simulink model "KUKA_PRRR"  (R2021a)
settings: Solver=FixedStepAuto  StartTime=0.0  StopTime=1  FixedStep=0.001  RelTol=1e-3
values from neighbouring files (symbols this model uses):
  m = {0 0 0 0 0}    [DynMatrixCalculator.m]    (also in DynMats_Iterative.mat = ; FinLagrange_2.m = mass{i})
  N = {zeros(3,1) zeros(3,1) zeros(3,1) zeros(3,1) zeros(3,1)}    [DynMatrixCalculator.m]    (also in DynMats_Iterative.mat = )
undefined symbols (not defined in the file or in its folder): X, Y, Z
libraries: sm_lib x17, nesl_utility x12
settings Model: Creator=Rahman Ardakanian  LastModifiedBy=Movazi
settings SolverCC: AlgebraicLoopSolver=TrustRegion
settings DebuggingCC: SFMachineParentedDataDiag=warning  ArithmeticOperatorsInVariantConditions=warning
settings SFSimCC: CustomCodeUndefinedFunction=UseInterfaceOnly
settings CodeAppCC: StateflowObjectComments=on

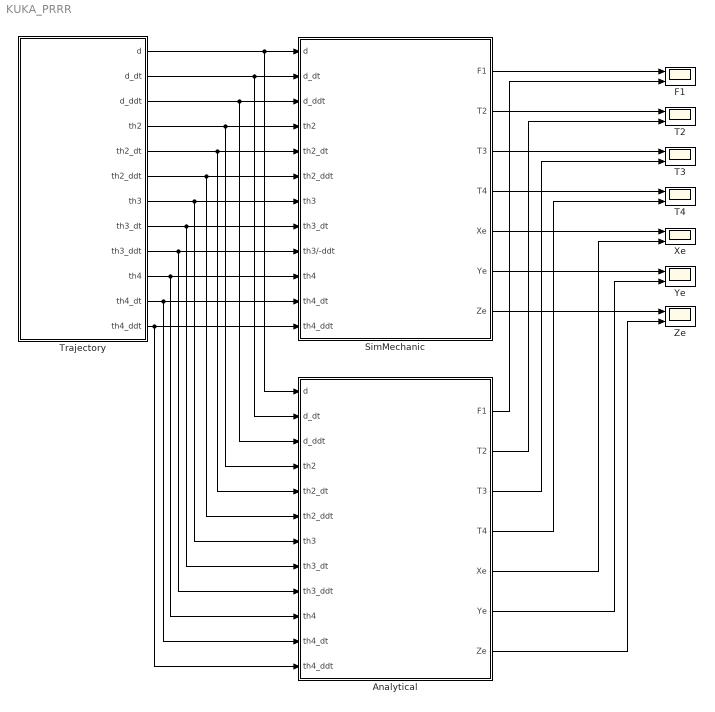
== system KUKA_PRRR ==
  Analytical : Subsystem
  F1 : Scope  NumInputPorts=2
  SimMechanic : Subsystem
  T2 : Scope  NumInputPorts=2
  T3 : Scope  NumInputPorts=2
  T4 : Scope  NumInputPorts=2
  Trajectory : Subsystem
  Xe : Scope  NumInputPorts=2
  Ye : Scope  NumInputPorts=2
  Ze : Scope  NumInputPorts=2
  wires:
  Trajectory/1(d) -> Analytical/1(d), SimMechanic/1(d)
  Trajectory/2(d_dt) -> Analytical/2(d_dt), SimMechanic/2(d_dt)
  Trajectory/3(d_ddt) -> Analytical/3(d_ddt), SimMechanic/3(d_ddt)
  Trajectory/4(th2) -> Analytical/4(th2), SimMechanic/4(th2)
  Trajectory/5(th2_dt) -> Analytical/5(th2_dt), SimMechanic/5(th2_dt)
  Trajectory/6(th2_ddt) -> Analytical/6(th2_ddt), SimMechanic/6(th2_ddt)
  Trajectory/7(th3) -> Analytical/7(th3), SimMechanic/7(th3)
  Trajectory/8(th3_dt) -> Analytical/8(th3_dt), SimMechanic/8(th3_dt)
  Trajectory/9(th3_ddt) -> Analytical/9(th3_ddt), SimMechanic/9(th3/-ddt)
  Trajectory/10(th4) -> Analytical/10(th4), SimMechanic/10(th4)
  Trajectory/11(th4_dt) -> Analytical/11(th4_dt), SimMechanic/11(th4_dt)
  Trajectory/12(th4_ddt) -> Analytical/12(th4_ddt), SimMechanic/12(th4_ddt)
  SimMechanic/1(F1) -> F1/1
  SimMechanic/2(T2) -> T2/1
  SimMechanic/3(T3) -> T3/1
  SimMechanic/4(T4) -> T4/1
  Analytical/1(F1) -> F1/2
  Analytical/2(T2) -> T2/2
  Analytical/3(T3) -> T3/2
  Analytical/4(T4) -> T4/2
  SimMechanic/5(Xe) -> Xe/1
  SimMechanic/6(Ye) -> Ye/1
  SimMechanic/7(Ze) -> Ze/1
  Analytical/5(Xe) -> Xe/2
  Analytical/6(Ye) -> Ye/2
  Analytical/7(Ze) -> Ze/2

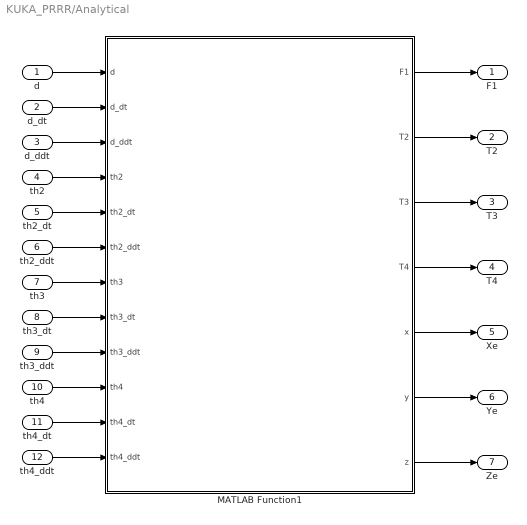
== system KUKA_PRRR/Analytical ==
  d : Inport
  d_dt : Inport  Port=2
  d_ddt : Inport  Port=3
  th2 : Inport  Port=4
  th2_dt : Inport  Port=5
  th2_ddt : Inport  Port=6
  th3 : Inport  Port=7
  th3_dt : Inport  Port=8
  th3_ddt : Inport  Port=9
  th4 : Inport  Port=10
  th4_dt : Inport  Port=11
  th4_ddt : Inport  Port=12
  MATLAB Function1 : MATLAB Function  TreatAsAtomicUnit=on
  F1 : Outport  VectorParamsAs1DForOutWhenUnconnected=off
  T2 : Outport  Port=2  VectorParamsAs1DForOutWhenUnconnected=off
  T3 : Outport  Port=3  VectorParamsAs1DForOutWhenUnconnected=off
  T4 : Outport  Port=4  VectorParamsAs1DForOutWhenUnconnected=off
  Xe : Outport  Port=5  VectorParamsAs1DForOutWhenUnconnected=off
  Ye : Outport  Port=6  VectorParamsAs1DForOutWhenUnconnected=off
  Ze : Outport  Port=7  VectorParamsAs1DForOutWhenUnconnected=off
  wires:
  MATLAB Function1/1(F1) -> F1/1
  d/1 -> MATLAB Function1/1(d)
  d_ddt/1 -> MATLAB Function1/3(d_ddt)
  d_dt/1 -> MATLAB Function1/2(d_dt)
  MATLAB Function1/4(T4) -> T4/1
  MATLAB Function1/3(T3) -> T3/1
  MATLAB Function1/2(T2) -> T2/1
  MATLAB Function1/5(x) -> Xe/1
  MATLAB Function1/6(y) -> Ye/1
  MATLAB Function1/7(z) -> Ze/1
  th2/1 -> MATLAB Function1/4(th2)
  th2_dt/1 -> MATLAB Function1/5(th2_dt)
  th2_ddt/1 -> MATLAB Function1/6(th2_ddt)
  th3/1 -> MATLAB Function1/7(th3)
  th3_dt/1 -> MATLAB Function1/8(th3_dt)
  th3_ddt/1 -> MATLAB Function1/9(th3_ddt)
  th4/1 -> MATLAB Function1/10(th4)
  th4_dt/1 -> MATLAB Function1/11(th4_dt)
  th4_ddt/1 -> MATLAB Function1/12(th4_ddt)

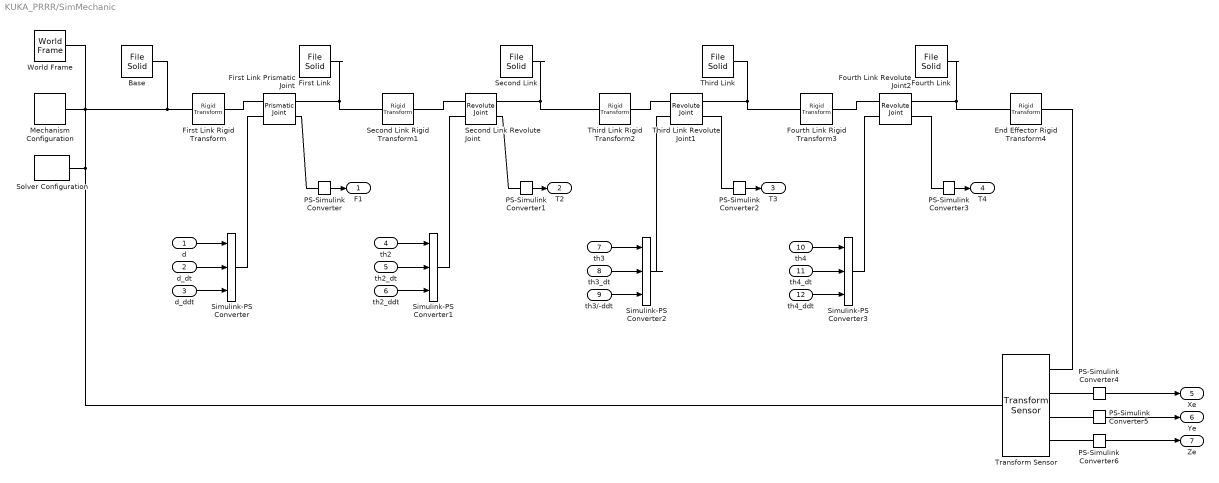
== system KUKA_PRRR/SimMechanic ==
  d : Inport
  d_dt : Inport  Port=2
  d_ddt : Inport  Port=3
  th2 : Inport  Port=4
  th2_dt : Inport  Port=5
  th2_ddt : Inport  Port=6
  th3 : Inport  Port=7
  th3_dt : Inport  Port=8
  th3/-ddt : Inport  Port=9
  th4 : Inport  Port=10
  th4_dt : Inport  Port=11
  th4_ddt : Inport  Port=12
  Base : sm_lib/Body Elements/File Solid  ExtGeomFileName=L0.STL  UnitType=Custom  ExtGeomFileUnits=mm  StepReaderType=HEX  ExportConvexHullGeometry=off  InertiaType=Custom  Mass=40.117  MassUnits=kg  CenterOfMass=[0 -0.033 0]  CenterOfMassUnits=m  MomentsOfInertia=[13.366 13.428 0.066]  MomentsOfInertiaUnits=kg*m^2  ProductsOfInertia=[0 0 0]  ProductsOfInertiaUnits=kg*m^2  BasedOnType=Density  Density=1000  DensityUnits=kg/m^3  DoExposeReferenceFrame=on  SerializedFrames=<Frames/>  GraphicType=FromGeometry  MarkerShape=Sphere  MarkerSize=10  GraphicVisPropType=SimpleVisualProperties  GraphicDiffuseColor=[0.5 0.5 0.5]  GraphicSpecularColor=[0.5 0.5 0.5 1.0]  GraphicAmbientColor=[0.15 0.15 0.15 1.0]  GraphicEmissiveColor=[0.0 0.0 0.0 1.0]  GraphicShininess=75  GraphicOpacity=1.0
  End Effector Rigid Transform4 : sm_lib/Frames and Transforms/Rigid Transform  TranslationMethod=Cartesian  TranslationStandardOffset=0  TranslationLengthUnit=mm  TranslationStandardAxis=+Z  TranslationCartesianOffset=[382.6 20 0]  TranslationROffset=0  TranslationROffsetUnits=m  TranslationZOffset=0  TranslationZOffsetUnits=m  TranslationThetaOffset=0  TranslationThetaOffsetUnits=deg  RotationMethod=AlignedAxes  RotationAngleUnits=deg  RotationStandardAxis=+Z  RotationAngle=0.0  RotationArbitraryAxis=[0 0 1]  FollAlignAxisA=+X  BaseAlignAxisA=+X  FollAlignAxisB=+Y  BaseAlignAxisB=+Y  RotationSequenceAxes=FollowerAxes  RotationSequence=XYX  RotationSequenceAngles=[0 0 0]  RotationSequenceAnglesUnits=deg  RotationMatrix=[1 0 0; 0 1 0; 0 0 1]
  First Link : sm_lib/Body Elements/File Solid  ExtGeomFileName=L1.STL  UnitType=Custom  ExtGeomFileUnits=mm  StepReaderType=HEX  ExportConvexHullGeometry=off  InertiaType=Custom  Mass=22.064  MassUnits=kg  CenterOfMass=[-0.031 0.094 0]  CenterOfMassUnits=m  MomentsOfInertia=[0.134 0.165 0.186]  MomentsOfInertiaUnits=kg*m^2  ProductsOfInertia=[0 0.001 -0.012]  ProductsOfInertiaUnits=kg*m^2  BasedOnType=Density  Density=1000  DensityUnits=kg/m^3  DoExposeReferenceFrame=on  SerializedFrames=<Frames/>  GraphicType=FromGeometry  MarkerShape=Sphere  MarkerSize=10  GraphicVisPropType=SimpleVisualProperties  GraphicDiffuseColor=[0.5 0.5 0.5]  GraphicSpecularColor=[0.5 0.5 0.5 1.0]  GraphicAmbientColor=[0.15 0.15 0.15 1.0]  GraphicEmissiveColor=[0.0 0.0 0.0 1.0]  GraphicShininess=75  GraphicOpacity=1.0
  First Link Prismatic Joint : sm_lib/Joints/Prismatic Joint  JointMode=Normal  SenseConstraintForce=off  SenseConstraintForceX=off  SenseConstraintForceY=off  SenseConstraintForceZ=off  SenseConstraintTorque=off  SenseConstraintTorqueX=off  SenseConstraintTorqueY=off  SenseConstraintTorqueZ=off  SenseTotalForce=off  SenseTotalForceX=off  SenseTotalForceY=off  SenseTotalForceZ=off  SenseTotalTorque=off  SenseTotalTorqueX=off  SenseTotalTorqueY=off  SenseTotalTorqueZ=off  CompositeWrenchDir=FollowerOnBase  CompositeWrenchFrame=BaseFrame  EquilibriumPosition=0  EquilibriumPositionUnits=m  SpringStiffness=0  SpringStiffnessUnits=N/m  DampingCoefficient=0  DampingCoefficientUnits=N/(m/s)  TorqueActuationMode=ComputedTorque  MotionActuationMode=InputMotion  SensePosition=off  SenseVelocity=off  SenseAcceleration=off  SenseTorqueForce=on  SenseLowerLimitTorqueForce=off  SenseUpperLimitTorqueForce=off  LowerLimitSpecify=off  LowerLimitBound=-1  LowerLimitBoundUnits=m  LowerLimitStiffness=1e6  LowerLimitStiffnessUnits=N/m  LowerLimitDamping=1e3  LowerLimitDampingUnits=N/(m/s)  LowerLimitTransitionRegionWidth=1e-4  LowerLimitTransitionRegionWidthUnits=m  UpperLimitSpecify=off  UpperLimitBound=1  UpperLimitBoundUnits=m  UpperLimitStiffness=1e6  UpperLimitStiffnessUnits=N/m  UpperLimitDamping=1e3  UpperLimitDampingUnits=N/(m/s)  UpperLimitTransitionRegionWidth=1e-4  UpperLimitTransitionRegionWidthUnits=m  PositionTargetSpecify=off  PositionTargetPriority=High  PositionTargetValue=0  PositionTargetValueUnits=m  VelocityTargetSpecify=off  VelocityTargetPriority=High  VelocityTargetValue=0  VelocityTargetValueUnits=m/s
  First Link Rigid Transform : sm_lib/Frames and Transforms/Rigid Transform  TranslationMethod=Cartesian  TranslationStandardOffset=0  TranslationLengthUnit=mm  TranslationStandardAxis=+Z  TranslationCartesianOffset=[0 0 0]  TranslationROffset=0  TranslationROffsetUnits=m  TranslationZOffset=0  TranslationZOffsetUnits=m  TranslationThetaOffset=0  TranslationThetaOffsetUnits=deg  RotationMethod=AlignedAxes  RotationAngleUnits=deg  RotationStandardAxis=+Z  RotationAngle=0.0  RotationArbitraryAxis=[0 0 1]  FollAlignAxisA=+X  BaseAlignAxisA=+X  FollAlignAxisB=+Y  BaseAlignAxisB=+Y  RotationSequenceAxes=FollowerAxes  RotationSequence=XYX  RotationSequenceAngles=[0 0 0]  RotationSequenceAnglesUnits=deg  RotationMatrix=[1 0 0; 0 1 0; 0 0 1]
  Fourth Link : sm_lib/Body Elements/File Solid  ExtGeomFileName=L4.STL  UnitType=Custom  ExtGeomFileUnits=mm  StepReaderType=HEX  ExportConvexHullGeometry=off  InertiaType=Custom  Mass=10.723  MassUnits=kg  CenterOfMass=[0.143 0.015 -0.001]  CenterOfMassUnits=m  MomentsOfInertia=[0.018 0.166 0.164]  MomentsOfInertiaUnits=kg*m^2  ProductsOfInertia=[0 -0.001 0.009]  ProductsOfInertiaUnits=kg*m^2  BasedOnType=Density  Density=1000  DensityUnits=kg/m^3  DoExposeReferenceFrame=on  SerializedFrames=<Frames/>  GraphicType=FromGeometry  MarkerShape=Sphere  MarkerSize=10  GraphicVisPropType=SimpleVisualProperties  GraphicDiffuseColor=[0.5 0.5 0.5]  GraphicSpecularColor=[0.5 0.5 0.5 1.0]  GraphicAmbientColor=[0.15 0.15 0.15 1.0]  GraphicEmissiveColor=[0.0 0.0 0.0 1.0]  GraphicShininess=75  GraphicOpacity=1.0
  Fourth Link Revolute Joint2 : sm_lib/Joints/Revolute Joint  JointMode=Normal  SenseConstraintForce=off  SenseConstraintForceX=off  SenseConstraintForceY=off  SenseConstraintForceZ=off  SenseConstraintTorque=off  SenseConstraintTorqueX=off  SenseConstraintTorqueY=off  SenseConstraintTorqueZ=off  SenseTotalForce=off  SenseTotalForceX=off  SenseTotalForceY=off  SenseTotalForceZ=off  SenseTotalTorque=off  SenseTotalTorqueX=off  SenseTotalTorqueY=off  SenseTotalTorqueZ=off  CompositeWrenchDir=FollowerOnBase  CompositeWrenchFrame=BaseFrame  EquilibriumPosition=0  EquilibriumPositionUnits=deg  SpringStiffness=0  SpringStiffnessUnits=N*m/deg  DampingCoefficient=0  DampingCoefficientUnits=N*m/(deg/s)  TorqueActuationMode=ComputedTorque  MotionActuationMode=InputMotion  SensePosition=off  SenseVelocity=off  SenseAcceleration=off  SenseTorqueForce=on  SenseLowerLimitTorqueForce=off  SenseUpperLimitTorqueForce=off  LowerLimitSpecify=off  LowerLimitBound=-90  LowerLimitBoundUnits=deg  LowerLimitStiffness=1e4  LowerLimitStiffnessUnits=N*m/deg  LowerLimitDamping=10  LowerLimitDampingUnits=N*m/(deg/s)  LowerLimitTransitionRegionWidth=0.1  LowerLimitTransitionRegionWidthUnits=deg  UpperLimitSpecify=off  UpperLimitBound=90  UpperLimitBoundUnits=deg  UpperLimitStiffness=1e4  UpperLimitStiffnessUnits=N*m/deg  UpperLimitDamping=10  UpperLimitDampingUnits=N*m/(deg/s)  UpperLimitTransitionRegionWidth=0.1  UpperLimitTransitionRegionWidthUnits=deg  PositionTargetSpecify=off  PositionTargetPriority=High  PositionTargetValue=0  PositionTargetValueUnits=deg  VelocityTargetSpecify=off  VelocityTargetPriority=High  VelocityTargetValue=0  VelocityTargetValueUnits=deg/s
  Fourth Link Rigid Transform3 : sm_lib/Frames and Transforms/Rigid Transform  TranslationMethod=Cartesian  TranslationStandardOffset=0  TranslationLengthUnit=mm  TranslationStandardAxis=+Z  TranslationCartesianOffset=[290 0 0]  TranslationROffset=0  TranslationROffsetUnits=m  TranslationZOffset=0  TranslationZOffsetUnits=m  TranslationThetaOffset=0  TranslationThetaOffsetUnits=deg  RotationMethod=AlignedAxes  RotationAngleUnits=deg  RotationStandardAxis=+Z  RotationAngle=0.0  RotationArbitraryAxis=[0 0 1]  FollAlignAxisA=+X  BaseAlignAxisA=-Y  FollAlignAxisB=+Z  BaseAlignAxisB=+Z  RotationSequenceAxes=FollowerAxes  RotationSequence=XYX  RotationSequenceAngles=[0 0 0]  RotationSequenceAnglesUnits=deg  RotationMatrix=[1 0 0; 0 1 0; 0 0 1]
  Mechanism Configuration : sm_lib/Utilities/Mechanism Configuration  UniformGravity=Constant  GravityVector=[0 -9.80665 0]  GravityVectorUnits=m/s^2  GravityUnits=m/s^2  LinearizationDelta=0.001  JointModeTransitionNonlinearIterations=2
  PS-Simulink Converter : nesl_utility/PS-Simulink Converter  PhysicalDomain=network_engine_domain  SubClassName=ps_output  LeftPortType=input  RightPortType=output  PseudoPeriodic=off  Frequencies=[]  Unit=N  AffineConversion=off
      settings: SourceProductBaseCode=PW,SS
  PS-Simulink Converter1 : nesl_utility/PS-Simulink Converter  PhysicalDomain=network_engine_domain  SubClassName=ps_output  LeftPortType=input  RightPortType=output  PseudoPeriodic=off  Frequencies=[]  Unit=N*m  AffineConversion=off
      settings: SourceProductBaseCode=PW,SS
  PS-Simulink Converter2 : nesl_utility/PS-Simulink Converter  PhysicalDomain=network_engine_domain  SubClassName=ps_output  LeftPortType=input  RightPortType=output  PseudoPeriodic=off  Frequencies=[]  Unit=N*m  AffineConversion=off
      settings: SourceProductBaseCode=PW,SS
  PS-Simulink Converter3 : nesl_utility/PS-Simulink Converter  PhysicalDomain=network_engine_domain  SubClassName=ps_output  LeftPortType=input  RightPortType=output  PseudoPeriodic=off  Frequencies=[]  Unit=N*m  AffineConversion=off
      settings: SourceProductBaseCode=PW,SS
  PS-Simulink Converter4 : nesl_utility/PS-Simulink Converter  PhysicalDomain=network_engine_domain  SubClassName=ps_output  LeftPortType=input  RightPortType=output  PseudoPeriodic=off  Frequencies=[]  Unit=m  AffineConversion=off
      settings: SourceProductBaseCode=PW,SS
  PS-Simulink Converter5 : nesl_utility/PS-Simulink Converter  PhysicalDomain=network_engine_domain  SubClassName=ps_output  LeftPortType=input  RightPortType=output  PseudoPeriodic=off  Frequencies=[]  Unit=m  AffineConversion=off
      settings: SourceProductBaseCode=PW,SS
  PS-Simulink Converter6 : nesl_utility/PS-Simulink Converter  PhysicalDomain=network_engine_domain  SubClassName=ps_output  LeftPortType=input  RightPortType=output  PseudoPeriodic=off  Frequencies=[]  Unit=m  AffineConversion=off
      settings: SourceProductBaseCode=PW,SS
  Second Link : sm_lib/Body Elements/File Solid  ExtGeomFileName=L2.STL  UnitType=Custom  ExtGeomFileUnits=mm  StepReaderType=HEX  ExportConvexHullGeometry=off  InertiaType=Custom  Mass=9.805  MassUnits=kg  CenterOfMass=[-0.005 -0.001 0.082]  CenterOfMassUnits=m  MomentsOfInertia=[0.082 0.053 0.058]  MomentsOfInertiaUnits=kg*m^2  ProductsOfInertia=[-0.001 0 0]  ProductsOfInertiaUnits=kg*m^2  BasedOnType=Density  Density=1000  DensityUnits=kg/m^3  DoExposeReferenceFrame=on  SerializedFrames=<Frames/>  GraphicType=FromGeometry  MarkerShape=Sphere  MarkerSize=10  GraphicVisPropType=SimpleVisualProperties  GraphicDiffuseColor=[0.5 0.5 0.5]  GraphicSpecularColor=[0.5 0.5 0.5 1.0]  GraphicAmbientColor=[0.15 0.15 0.15 1.0]  GraphicEmissiveColor=[0.0 0.0 0.0 1.0]  GraphicShininess=75  GraphicOpacity=1.0
  Second Link Revolute Joint : sm_lib/Joints/Revolute Joint  JointMode=Normal  SenseConstraintForce=off  SenseConstraintForceX=off  SenseConstraintForceY=off  SenseConstraintForceZ=off  SenseConstraintTorque=off  SenseConstraintTorqueX=off  SenseConstraintTorqueY=off  SenseConstraintTorqueZ=off  SenseTotalForce=off  SenseTotalForceX=off  SenseTotalForceY=off  SenseTotalForceZ=off  SenseTotalTorque=off  SenseTotalTorqueX=off  SenseTotalTorqueY=off  SenseTotalTorqueZ=off  CompositeWrenchDir=FollowerOnBase  CompositeWrenchFrame=BaseFrame  EquilibriumPosition=0  EquilibriumPositionUnits=deg  SpringStiffness=0  SpringStiffnessUnits=N*m/deg  DampingCoefficient=0  DampingCoefficientUnits=N*m/(deg/s)  TorqueActuationMode=ComputedTorque  MotionActuationMode=InputMotion  SensePosition=off  SenseVelocity=off  SenseAcceleration=off  SenseTorqueForce=on  SenseLowerLimitTorqueForce=off  SenseUpperLimitTorqueForce=off  LowerLimitSpecify=off  LowerLimitBound=-90  LowerLimitBoundUnits=deg  LowerLimitStiffness=1e4  LowerLimitStiffnessUnits=N*m/deg  LowerLimitDamping=10  LowerLimitDampingUnits=N*m/(deg/s)  LowerLimitTransitionRegionWidth=0.1  LowerLimitTransitionRegionWidthUnits=deg  UpperLimitSpecify=off  UpperLimitBound=90  UpperLimitBoundUnits=deg  UpperLimitStiffness=1e4  UpperLimitStiffnessUnits=N*m/deg  UpperLimitDamping=10  UpperLimitDampingUnits=N*m/(deg/s)  UpperLimitTransitionRegionWidth=0.1  UpperLimitTransitionRegionWidthUnits=deg  PositionTargetSpecify=off  PositionTargetPriority=High  PositionTargetValue=0  PositionTargetValueUnits=deg  VelocityTargetSpecify=off  VelocityTargetPriority=High  VelocityTargetValue=0  VelocityTargetValueUnits=deg/s
  Second Link Rigid Transform1 : sm_lib/Frames and Transforms/Rigid Transform  TranslationMethod=Cartesian  TranslationStandardOffset=0  TranslationLengthUnit=mm  TranslationStandardAxis=+Z  TranslationCartesianOffset=[0 197 0]  TranslationROffset=0  TranslationROffsetUnits=m  TranslationZOffset=0  TranslationZOffsetUnits=m  TranslationThetaOffset=0  TranslationThetaOffsetUnits=deg  RotationMethod=AlignedAxes  RotationAngleUnits=deg  RotationStandardAxis=+Z  RotationAngle=0.0  RotationArbitraryAxis=[0 0 1]  FollAlignAxisA=+X  BaseAlignAxisA=+X  FollAlignAxisB=+Y  BaseAlignAxisB=-Z  RotationSequenceAxes=FollowerAxes  RotationSequence=XYX  RotationSequenceAngles=[0 0 0]  RotationSequenceAnglesUnits=deg  RotationMatrix=[1 0 0; 0 1 0; 0 0 1]
  Simulink-PS Converter : nesl_utility/Simulink-PS Converter  PhysicalDomain=network_engine_domain  SubClassName=ps_input  LeftPortType=input  RightPortType=output  PseudoPeriodic=off  Frequencies=[]  NoiseDistribution=none  NoiseParameters=[]  Unit=m  AffineConversion=off  FilteringAndDerivatives=provide  SimscapeFilterOrder=1  InputFilterTimeConstant=0.001  UdotUserProvided=2
      settings: SourceProductBaseCode=PW,SS
  Simulink-PS Converter1 : nesl_utility/Simulink-PS Converter  PhysicalDomain=network_engine_domain  SubClassName=ps_input  LeftPortType=input  RightPortType=output  PseudoPeriodic=off  Frequencies=[]  NoiseDistribution=none  NoiseParameters=[]  Unit=rad  AffineConversion=off  FilteringAndDerivatives=provide  SimscapeFilterOrder=1  InputFilterTimeConstant=0.001  UdotUserProvided=2
      settings: SourceProductBaseCode=PW,SS
  Simulink-PS Converter2 : nesl_utility/Simulink-PS Converter  PhysicalDomain=network_engine_domain  SubClassName=ps_input  LeftPortType=input  RightPortType=output  PseudoPeriodic=off  Frequencies=[]  NoiseDistribution=none  NoiseParameters=[]  Unit=rad  AffineConversion=off  FilteringAndDerivatives=provide  SimscapeFilterOrder=1  InputFilterTimeConstant=0.001  UdotUserProvided=2
      settings: SourceProductBaseCode=PW,SS
  Simulink-PS Converter3 : nesl_utility/Simulink-PS Converter  PhysicalDomain=network_engine_domain  SubClassName=ps_input  LeftPortType=input  RightPortType=output  PseudoPeriodic=off  Frequencies=[]  NoiseDistribution=none  NoiseParameters=[]  Unit=rad  AffineConversion=off  FilteringAndDerivatives=provide  SimscapeFilterOrder=1  InputFilterTimeConstant=0.001  UdotUserProvided=2
      settings: SourceProductBaseCode=PW,SS
  Solver Configuration : nesl_utility/Solver Configuration  PhysicalDomain=network_engine_domain  SubClassName=solver  LeftPortType=input  RightPortType=generic  Tones=[]  Harmonics=[]  SimulateNoise=off  Profile=off  UseLocalSampling=off  EnableSwitchedLinearOptims=on  FrequencyDomain=off  UseCCode=off  RelTol=0.001  AbsTol=1e-06  MinStep=1e-09  ToWorkspace=off  RevertToSquareIcSolve=off  NumHomotopyIterations=100  PhasorMode=off  PhasorModeNumHarmonics=1  DoDC=off  ResidualTolerance=1e-09  UseLocalSolver=off  LocalSolverChoice=NE_BACKWARD_EULER_ADVANCER  LocalSolverSampleTime=0.001  DoFixedCost=off  MaxNonlinIter=3  MaxModeIter=2  ComputeImpulses=off  ImpulseIterations=2  LinearAlgebra=Sparse  EquationFormulation=NE_TIME_EF  DelaysMemoryBudget=1024  AutomaticFiltering=on  FilteringTimeConstant=0.001  PartitionStorageMethod=AS_NEEDED  PartitionMemoryBudget=1024  PartitionMethod=FAST
      settings: SourceProductBaseCode=PW,SS
  Third Link : sm_lib/Body Elements/File Solid  ExtGeomFileName=L3.STL  UnitType=Custom  ExtGeomFileUnits=mm  StepReaderType=HEX  ExportConvexHullGeometry=off  InertiaType=Custom  Mass=13.302  MassUnits=kg  CenterOfMass=[0.118 0.011 -0.001]  CenterOfMassUnits=m  MomentsOfInertia=[0.048 0.176 0.154]  MomentsOfInertiaUnits=kg*m^2  ProductsOfInertia=[0 0.002 0.003]  ProductsOfInertiaUnits=kg*m^2  BasedOnType=Density  Density=1000  DensityUnits=kg/m^3  DoExposeReferenceFrame=on  SerializedFrames=<Frames/>  GraphicType=FromGeometry  MarkerShape=Sphere  MarkerSize=10  GraphicVisPropType=SimpleVisualProperties  GraphicDiffuseColor=[0.5 0.5 0.5]  GraphicSpecularColor=[0.5 0.5 0.5 1.0]  GraphicAmbientColor=[0.15 0.15 0.15 1.0]  GraphicEmissiveColor=[0.0 0.0 0.0 1.0]  GraphicShininess=75  GraphicOpacity=1.0
  Third Link Revolute Joint1 : sm_lib/Joints/Revolute Joint  JointMode=Normal  SenseConstraintForce=off  SenseConstraintForceX=off  SenseConstraintForceY=off  SenseConstraintForceZ=off  SenseConstraintTorque=off  SenseConstraintTorqueX=off  SenseConstraintTorqueY=off  SenseConstraintTorqueZ=off  SenseTotalForce=off  SenseTotalForceX=off  SenseTotalForceY=off  SenseTotalForceZ=off  SenseTotalTorque=off  SenseTotalTorqueX=off  SenseTotalTorqueY=off  SenseTotalTorqueZ=off  CompositeWrenchDir=FollowerOnBase  CompositeWrenchFrame=BaseFrame  EquilibriumPosition=0  EquilibriumPositionUnits=deg  SpringStiffness=0  SpringStiffnessUnits=N*m/deg  DampingCoefficient=0  DampingCoefficientUnits=N*m/(deg/s)  TorqueActuationMode=ComputedTorque  MotionActuationMode=InputMotion  SensePosition=off  SenseVelocity=off  SenseAcceleration=off  SenseTorqueForce=on  SenseLowerLimitTorqueForce=off  SenseUpperLimitTorqueForce=off  LowerLimitSpecify=off  LowerLimitBound=-90  LowerLimitBoundUnits=deg  LowerLimitStiffness=1e4  LowerLimitStiffnessUnits=N*m/deg  LowerLimitDamping=10  LowerLimitDampingUnits=N*m/(deg/s)  LowerLimitTransitionRegionWidth=0.1  LowerLimitTransitionRegionWidthUnits=deg  UpperLimitSpecify=off  UpperLimitBound=90  UpperLimitBoundUnits=deg  UpperLimitStiffness=1e4  UpperLimitStiffnessUnits=N*m/deg  UpperLimitDamping=10  UpperLimitDampingUnits=N*m/(deg/s)  UpperLimitTransitionRegionWidth=0.1  UpperLimitTransitionRegionWidthUnits=deg  PositionTargetSpecify=off  PositionTargetPriority=High  PositionTargetValue=0  PositionTargetValueUnits=deg  VelocityTargetSpecify=off  VelocityTargetPriority=High  VelocityTargetValue=0  VelocityTargetValueUnits=deg/s
  Third Link Rigid Transform2 : sm_lib/Frames and Transforms/Rigid Transform  TranslationMethod=Cartesian  TranslationStandardOffset=0  TranslationLengthUnit=mm  TranslationStandardAxis=+Z  TranslationCartesianOffset=[0 0 152.5]  TranslationROffset=0  TranslationROffsetUnits=m  TranslationZOffset=0  TranslationZOffsetUnits=m  TranslationThetaOffset=0  TranslationThetaOffsetUnits=deg  RotationMethod=AlignedAxes  RotationAngleUnits=deg  RotationStandardAxis=+Z  RotationAngle=0.0  RotationArbitraryAxis=[0 0 1]  FollAlignAxisA=+X  BaseAlignAxisA=+Z  FollAlignAxisB=+Z  BaseAlignAxisB=-Y  RotationSequenceAxes=FollowerAxes  RotationSequence=XYX  RotationSequenceAngles=[0 0 0]  RotationSequenceAnglesUnits=deg  RotationMatrix=[1 0 0; 0 1 0; 0 0 1]
  Transform Sensor : sm_lib/Frames and Transforms/Transform Sensor  MeasurementFrame=World  SenseAngle=off  SenseAxis=off  SenseAngle1=off  SenseAngle2=off  SenseAngle3=off  SenseQ=off  SenseR=off  SenseOmegaX=off  SenseOmegaY=off  SenseOmegaZ=off  SenseOmega1=off  SenseOmega2=off  SenseOmega3=off  SenseQDot=off  SenseRDot=off  SenseAlphaX=off  SenseAlphaY=off  SenseAlphaZ=off  SenseAlpha1=off  SenseAlpha2=off  SenseAlpha3=off  SenseQDDot=off  SenseRDDot=off  SenseX=on  SenseY=on  SenseZ=on  SenseRad=off  SenseAzim=off  SenseDist=off  SenseInc=off  SenseXDot=off  SenseYDot=off  SenseZDot=off  SenseRadDot=off  SenseAzimDot=off  SenseDistDot=off  SenseIncDot=off  SenseXDDot=off  SenseYDDot=off  SenseZDDot=off  SenseRadDDot=off  SenseAzimDDot=off  SenseDistDDot=off  SenseIncDDot=off
  World Frame : sm_lib/Frames and Transforms/World Frame
  F1 : Outport  VectorParamsAs1DForOutWhenUnconnected=off
  T2 : Outport  Port=2  VectorParamsAs1DForOutWhenUnconnected=off
  T3 : Outport  Port=3  VectorParamsAs1DForOutWhenUnconnected=off
  T4 : Outport  Port=4  VectorParamsAs1DForOutWhenUnconnected=off
  Xe : Outport  Port=5  VectorParamsAs1DForOutWhenUnconnected=off
  Ye : Outport  Port=6  VectorParamsAs1DForOutWhenUnconnected=off
  Ze : Outport  Port=7  VectorParamsAs1DForOutWhenUnconnected=off
  wires:
  d/1 -> Simulink-PS Converter/1
  d_ddt/1 -> Simulink-PS Converter/3
  d_dt/1 -> Simulink-PS Converter/2
  PS-Simulink Converter/1 -> F1/1
  PS-Simulink Converter1/1 -> T2/1
  th2_dt/1 -> Simulink-PS Converter1/2
  th2_ddt/1 -> Simulink-PS Converter1/3
  th2/1 -> Simulink-PS Converter1/1
  th3/1 -> Simulink-PS Converter2/1
  th3/-ddt/1 -> Simulink-PS Converter2/3
  th3_dt/1 -> Simulink-PS Converter2/2
  PS-Simulink Converter2/1 -> T3/1
  PS-Simulink Converter3/1 -> T4/1
  th4_dt/1 -> Simulink-PS Converter3/2
  th4_ddt/1 -> Simulink-PS Converter3/3
  th4/1 -> Simulink-PS Converter3/1
  PS-Simulink Converter4/1 -> Xe/1
  PS-Simulink Converter5/1 -> Ye/1
  PS-Simulink Converter6/1 -> Ze/1
  connections:
  End Effector Rigid Transform4/LConn1 -- Fourth Link/RConn1 -- Fourth Link Revolute Joint2/RConn1
  Third Link Rigid Transform2/LConn1 -- Second Link/RConn1 -- Second Link Revolute Joint/RConn1
  World Frame/RConn1 -- Transform Sensor/LConn1 -- Solver Configuration/RConn1 -- First Link Rigid Transform/LConn1 -- Base/RConn1 -- Mechanism Configuration/RConn1
  Third Link Revolute Joint1/RConn1 -- Fourth Link Rigid Transform3/LConn1 -- Third Link/RConn1
  First Link Prismatic Joint/LConn1 -- First Link Rigid Transform/RConn1
  Fourth Link Revolute Joint2/LConn1 -- Fourth Link Rigid Transform3/RConn1
  Second Link Rigid Transform1/LConn1 -- First Link/RConn1 -- First Link Prismatic Joint/RConn1
  Third Link Revolute Joint1/LConn1 -- Third Link Rigid Transform2/RConn1
  Second Link Revolute Joint/LConn1 -- Second Link Rigid Transform1/RConn1
  Transform Sensor/RConn1 -- End Effector Rigid Transform4/RConn1
  Simulink-PS Converter/RConn1 -- First Link Prismatic Joint/LConn2
  PS-Simulink Converter/LConn1 -- First Link Prismatic Joint/RConn2
  PS-Simulink Converter1/LConn1 -- Second Link Revolute Joint/RConn2
  Simulink-PS Converter1/RConn1 -- Second Link Revolute Joint/LConn2
  Simulink-PS Converter2/RConn1 -- Third Link Revolute Joint1/LConn2
  PS-Simulink Converter2/LConn1 -- Third Link Revolute Joint1/RConn2
  PS-Simulink Converter3/LConn1 -- Fourth Link Revolute Joint2/RConn2
  Simulink-PS Converter3/RConn1 -- Fourth Link Revolute Joint2/LConn2
  PS-Simulink Converter4/LConn1 -- Transform Sensor/RConn2
  PS-Simulink Converter5/LConn1 -- Transform Sensor/RConn3
  PS-Simulink Converter6/LConn1 -- Transform Sensor/RConn4

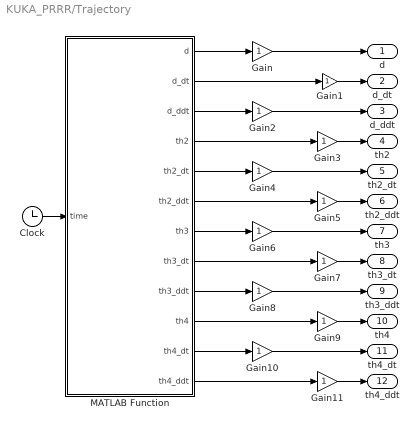
== system KUKA_PRRR/Trajectory ==
  Clock : Clock
  Gain{,1..11} (12 alike) : Gain
  MATLAB Function : MATLAB Function  TreatAsAtomicUnit=on
  d : Outport  VectorParamsAs1DForOutWhenUnconnected=off
  d_dt : Outport  Port=2  VectorParamsAs1DForOutWhenUnconnected=off
  d_ddt : Outport  Port=3  VectorParamsAs1DForOutWhenUnconnected=off
  th2 : Outport  Port=4  VectorParamsAs1DForOutWhenUnconnected=off
  th2_dt : Outport  Port=5  VectorParamsAs1DForOutWhenUnconnected=off
  th2_ddt : Outport  Port=6  VectorParamsAs1DForOutWhenUnconnected=off
  th3 : Outport  Port=7  VectorParamsAs1DForOutWhenUnconnected=off
  th3_dt : Outport  Port=8  VectorParamsAs1DForOutWhenUnconnected=off
  th3_ddt : Outport  Port=9  VectorParamsAs1DForOutWhenUnconnected=off
  th4 : Outport  Port=10  VectorParamsAs1DForOutWhenUnconnected=off
  th4_dt : Outport  Port=11  VectorParamsAs1DForOutWhenUnconnected=off
  th4_ddt : Outport  Port=12  VectorParamsAs1DForOutWhenUnconnected=off
  wires:
  Clock/1 -> MATLAB Function/1(time)
  MATLAB Function/1(d) -> Gain/1
  MATLAB Function/2(d_dt) -> Gain1/1
  MATLAB Function/3(d_ddt) -> Gain2/1
  MATLAB Function/4(th2) -> Gain3/1
  MATLAB Function/5(th2_dt) -> Gain4/1
  MATLAB Function/6(th2_ddt) -> Gain5/1
  MATLAB Function/7(th3) -> Gain6/1
  MATLAB Function/8(th3_dt) -> Gain7/1
  MATLAB Function/9(th3_ddt) -> Gain8/1
  MATLAB Function/10(th4) -> Gain9/1
  MATLAB Function/11(th4_dt) -> Gain10/1
  MATLAB Function/12(th4_ddt) -> Gain11/1
  Gain/1 -> d/1
  Gain1/1 -> d_dt/1
  Gain2/1 -> d_ddt/1
  Gain3/1 -> th2/1
  Gain4/1 -> th2_dt/1
  Gain5/1 -> th2_ddt/1
  Gain6/1 -> th3/1
  Gain7/1 -> th3_dt/1
  Gain8/1 -> th3_ddt/1
  Gain9/1 -> th4/1
  Gain10/1 -> th4_dt/1
  Gain11/1 -> th4_ddt/1

== matlab function KUKA_PRRR/Analytical/MATLAB Function1 ==
  data: d input; F1 output; d_dt input; d_ddt input; th2 input; th2_dt input; th2_ddt input; th3 input; th3_dt input; th3_ddt input; th4 input; th4_dt input; th4_ddt input; T2 output; T3 output; T4 output; x output; y output; z output
function [F1,T2,T3,T4,x,y,z] = fcn(d,d_dt,d_ddt,th2,th2_dt,th2_ddt,th3,th3_dt,th3_ddt,th4,th4_dt,th4_ddt)

%mass of links
g=9.80665;
m0=40.117;
m{1}=22.064;
m{2}=9.805;
m{3}=13.302;
m{4}=10.723;
% center of mass in it's cordination
Pc0=[0;-0.033;0];
Pc{1}=[-0.031;0.165;0.186];
Pc{2}=[-0.005;-0.001;0.082];
Pc{3}=[0.118;0.011;-0.001];
Pc{4}=[0.143;0.015;-0.001];
% moment inertia of links in their cordinations
I0=[13.366 0 0;0 13.428 0;0 0 0.066];
I{1}=[0.134 -0.012 0.001;-0.012 0.165 0;0.001 0 0.186];
I{2}=[0.082 0 0;0 0.053 -0.001;0 -0.001 0.058];
I{3}=[0.048 0.003 0.002;0.003 0.176 0;0.002 0 0.154];
I{4}=[0.018 0.009 -0.001;0.009 0.166 0;-0.001 0 0.164];
% Rotation matrixes
R{1}=[1 0 0;0 1 0;0 0 1];
R{2}=[cos(th2) -sin(th2) 0;0 0 1;-sin(th2) -cos(th2) 0];
R{3}=[-sin(th3) -cos(th3) 0;0 0 -1;cos(th3) -sin(th3) 0];
R{4}=[sin(th4) cos(th4) 0;-cos(th4) sin(th4) 0;0 0 1];
R{5}=[1 0 0;0 1 0;0 0 1];
% each cordination in pervious coordination
P0=[0;0;0];
P{1}=[0;0;d];
P{2}=[0;0.197;0];
P{3}=[0;0;0.1525];
P{4}=[0.290;0;0];
P{5}=[0.3826;0.020;0];

M =[                                                                                                                                                                                                                                                                                                                                                       27947/500, (1961*cos(th2))/40000 + (711*sin(th2))/50000 + (2339653*cos(th2)*sin(th3))/500000 + (73161*cos(th2)*cos(th3))/500000 - (1533389*cos(th2)*cos(th3)*cos(th4))/1000000 + (32169*cos(th2)*cos(th3)*sin(th4))/200000 + (32169*cos(th2)*cos(th4)*sin(th3))/200000 + (1533389*cos(th2)*sin(th3)*sin(th4))/1000000,  sin(th2)*((5479328692330^(1/2)*cos(atan(73161/2339653) + th3))/500000 + (10723*20674^(1/2)*sin(atan(15/143) + th3 + th4))/1000000),     (10723*20674^(1/2)*sin(atan(15/143) + th3 + th4)*sin(th2))/1000000
    (1961*cos(th2))/40000 + (711*sin(th2))/50000 + (2339653*cos(th2)*sin(th3))/500000 + (73161*cos(th2)*cos(th3))/500000 - (1533389*cos(th2)*cos(th3)*cos(th4))/1000000 + (32169*cos(th2)*cos(th3)*sin(th4))/200000 + (32169*cos(th2)*cos(th4)*sin(th3))/200000 + (1533389*cos(th2)*sin(th3)*sin(th4))/1000000,                                (310967*20674^(1/2)*cos(atan(143/15) - th4))/100000000 - (310967*20674^(1/2)*cos(2*th3 - atan(143/15) + th4))/100000000 - (3*1636869206119633^(1/2)*cos(atan(4755332/202235301) + 2*th3))/200000000 + (33477084385009801^(1/2)*cos(atan(14000835/182430976) + 2*th3 + 2*th4))/1000000000 + 917438051/1000000000, (310374939346^(1/2)*cos(th3 - atan(533389/160845) + th4))/1000000000 + (11158634692330^(1/2)*cos(atan(73161/3339653) + th3))/500000000,      (310374939346^(1/2)*sin(atan(160845/533389) + th3 + th4))/1000000000
    (sin(th2)*(2*5479328692330^(1/2)*cos(atan(73161/2339653) + th3) + 10723*20674^(1/2)*sin(atan(15/143) + th3 + th4)))/1000000,                                                                                                                                                                                                                  (310374939346^(1/2)*cos(th3 - atan(533389/160845) + th4))/1000000000 + (11158634692330^(1/2)*cos(atan(73161/3339653) + th3))/500000000,                                                                   (310967*20674^(1/2)*cos(atan(143/15) - th4))/50000000 + 101769887/62500000, (310967*20674^(1/2)*cos(atan(143/15) - th4))/100000000 + 192843651/500000000
    (10723*20674^(1/2)*sin(atan(15/143) + th3 + th4)*sin(th2))/1000000,                                                                                                                                                                                                                                                                                       (310374939346^(1/2)*cos(th3 - atan(533389/160845) + th4))/1000000000,                                                                 (310967*20674^(1/2)*cos(atan(143/15) - th4))/100000000 + 192843651/500000000,                                                             192843651/500000000];

V =[(711*cos(th2)*th2_dt^2)/50000 - (1961*sin(th2)*th2_dt^2)/40000 - (73161*cos(th3)*sin(th2)*th2_dt^2)/500000 - (73161*cos(th3)*sin(th2)*th3_dt^2)/500000 - (2339653*sin(th2)*sin(th3)*th2_dt^2)/500000 - (2339653*sin(th2)*sin(th3)*th3_dt^2)/500000 + (1533389*cos(th3)*cos(th4)*sin(th2)*th2_dt^2)/1000000 + (1533389*cos(th3)*cos(th4)*sin(th2)*th3_dt^2)/1000000 + (1533389*cos(th3)*cos(th4)*sin(th2)*th4_dt^2)/1000000 + (2339653*cos(th2)*cos(th3)*th2_dt*th3_dt)/250000 - (32169*cos(th3)*sin(th2)*sin(th4)*th2_dt^2)/200000 - (32169*cos(th4)*sin(th2)*sin(th3)*th2_dt^2)/200000 - (32169*cos(th3)*sin(th2)*sin(th4)*th3_dt^2)/200000 - (32169*cos(th4)*sin(th2)*sin(th3)*th3_dt^2)/200000 - (32169*cos(th3)*sin(th2)*sin(th4)*th4_dt^2)/200000 - (32169*cos(th4)*sin(th2)*sin(th3)*th4_dt^2)/200000 - (73161*cos(th2)*sin(th3)*th2_dt*th3_dt)/250000 - (1533389*sin(th2)*sin(th3)*sin(th4)*th2_dt^2)/1000000 - (1533389*sin(th2)*sin(th3)*sin(th4)*th3_dt^2)/1000000 - (1533389*sin(th2)*sin(th3)*sin(th4)*th4_dt^2)/1000000 + (32169*cos(th2)*cos(th3)*cos(th4)*th2_dt*th3_dt)/100000 + (32169*cos(th2)*cos(th3)*cos(th4)*th2_dt*th4_dt)/100000 + (1533389*cos(th2)*cos(th3)*sin(th4)*th2_dt*th3_dt)/500000 + (1533389*cos(th2)*cos(th4)*sin(th3)*th2_dt*th3_dt)/500000 + (1533389*cos(th2)*cos(th3)*sin(th4)*th2_dt*th4_dt)/500000 + (1533389*cos(th2)*cos(th4)*sin(th3)*th2_dt*th4_dt)/500000 + (1533389*cos(th3)*cos(th4)*sin(th2)*th3_dt*th4_dt)/500000 - (32169*cos(th2)*sin(th3)*sin(th4)*th2_dt*th3_dt)/100000 - (32169*cos(th2)*sin(th3)*sin(th4)*th2_dt*th4_dt)/100000 - (32169*cos(th3)*sin(th2)*sin(th4)*th3_dt*th4_dt)/100000 - (32169*cos(th4)*sin(th2)*sin(th3)*th3_dt*th4_dt)/100000 - (1533389*sin(th2)*sin(th3)*sin(th4)*th3_dt*th4_dt)/500000
    (533389*cos(th3 + th4)*th3_dt^2)/1000000000 + (533389*cos(th3 + th4)*th4_dt^2)/1000000000 - (32169*sin(th3 + th4)*th3_dt^2)/200000000 - (32169*sin(th3 + th4)*th4_dt^2)/200000000 - (73161*cos(th3)*th3_dt^2)/500000000 - (3339653*sin(th3)*th3_dt^2)/500000000 + (44468281*cos(th4)*th2_dt*th4_dt)/100000000 - (2800167*cos(2*th3 + 2*th4)*th2_dt*th3_dt)/100000000 - (2800167*cos(2*th3 + 2*th4)*th2_dt*th4_dt)/100000000 - (932901*sin(th4)*th2_dt*th4_dt)/20000000 - (712621*sin(2*th3 + 2*th4)*th2_dt*th3_dt)/1953125 - (712621*sin(2*th3 + 2*th4)*th2_dt*th4_dt)/1953125 + (533389*cos(th3 + th4)*th3_dt*th4_dt)/500000000 - (32169*sin(th3 + th4)*th3_dt*th4_dt)/100000000 + (3566499*cos(2*th3)*th2_dt*th3_dt)/125000000 + (606705903*sin(2*th3)*th2_dt*th3_dt)/500000000 - (44468281*cos(2*th3 + th4)*th2_dt*th3_dt)/50000000 - (44468281*cos(2*th3 + th4)*th2_dt*th4_dt)/100000000 + (932901*sin(2*th3 + th4)*th2_dt*th3_dt)/10000000 + (932901*sin(2*th3 + th4)*th2_dt*th4_dt)/20000000
    (44468281*cos(2*th3 + th4)*th2_dt^2)/100000000 - (606705903*sin(2*th3)*th2_dt^2)/1000000000 - (3566499*cos(2*th3)*th2_dt^2)/250000000 - (932901*sin(2*th3 + th4)*th2_dt^2)/20000000 + (44468281*cos(th4)*th4_dt^2)/100000000 + (2800167*cos(2*th3 + 2*th4)*th2_dt^2)/200000000 - (932901*sin(th4)*th4_dt^2)/20000000 + (712621*sin(2*th3 + 2*th4)*th2_dt^2)/3906250 + (44468281*cos(th4)*th3_dt*th4_dt)/50000000 - (932901*sin(th4)*th3_dt*th4_dt)/10000000
    (44468281*cos(2*th3 + th4)*th2_dt^2)/200000000 - (932901*sin(2*th3 + th4)*th2_dt^2)/40000000 - (44468281*cos(th4)*th2_dt^2)/200000000 - (44468281*cos(th4)*th3_dt^2)/100000000 + (2800167*cos(2*th3 + 2*th4)*th2_dt^2)/200000000 + (932901*sin(th4)*th2_dt^2)/40000000 + (932901*sin(th4)*th3_dt^2)/20000000 + (712621*sin(2*th3 + 2*th4)*th2_dt^2)/3906250];
G =[                                                                                                                                               0
    0
    (1533389*g*cos(th3 + th4))/1000000 - (2339653*g*sin(th3))/500000 - (73161*g*cos(th3))/500000 - (32169*g*sin(th3 + th4))/200000
    (1533389*g*cos(th3 + th4))/1000000 - (32169*g*sin(th3 + th4))/200000];

EEP=P{1}+R{1}*P{2}+R{1}*R{2}*P{3}+R{1}*R{2}*R{3}*P{4}+R{1}*R{2}*R{3}*R{4}*P{5};
FT=M*[d_ddt;th2_ddt;th3_ddt;th4_ddt]+V+G;

F1=FT(1);T2=FT(2);T3=FT(3);T4=T(4);
x=EEP(1);y=EEP(2);z=EEP(3);
end

== matlab function KUKA_PRRR/Trajectory/MATLAB Function ==
  data: time input; d output; d_dt output; d_ddt output; th2 output; th2_dt output; th2_ddt output; th3 output; th3_dt output; th3_ddt output; th4 output; th4_dt output; th4_ddt output
function [d,d_dt,d_ddt,th2,th2_dt,th2_ddt,th3,th3_dt,th3_ddt,th4,th4_dt,th4_ddt] = fcn(time)
time=time*5;
d=  (1/4)*(1-cos(time*pi/5));
th2= (pi/4)*(1-cos(time*pi/5));
th3= -(pi/4)*(1-cos(time*pi/5));
th4=  (pi/4)*(1-cos(time*pi/5));

d_dt= (pi/20)*sin(time*pi/5);
th2_dt=(pi^2/20)*sin(time*pi/5);
th3_dt=-(pi^2/20)*sin(time*pi/5);
th4_dt= (pi^2/20)*sin(time*pi/5);

d_ddt= (pi^2/100)*cos(time*pi/5);
th2_ddt=(pi^3/100)*cos(time*pi/5);
th3_ddt=-(pi^3/100)*cos(time*pi/5);
th4_ddt= (pi^3/100)*cos(time*pi/5);
